simulink model "gsm_ddc_model"  (R2025a)
settings: Solver=VariableStepAuto  StartTime=0.0  StopTime=3  FixedStep=0.00005  RelTol=1e-3
undefined symbols (not defined in the file): designMultirateFIR, dspblkCoreblockFVToolHelper, gcbh
libraries: dspmlti4 x10, dspsigops x8, dspsrcs4 x8
settings Model: Creator=User  LastModifiedBy=User
settings OptimizationCC: DefaultParameterBehavior=Inlined  EnhancedBackFolding=on  PassReuseOutputArgsAs=Individual arguments  ZeroExternalMemoryAtStartup=off  ZeroInternalMemoryAtStartup=off  OptimizeBlockOrder=speed  DifferentSizesBufferReuse=on  OptimizationCustomize=off  EfficientTunableParamExpr=on
settings DebuggingCC: ParameterTunabilityLossMsg=error
settings HardwareCC: TargetBitPerPointer=64.0  TargetBitPerSizeT=64.0  TargetBitPerPtrDiffT=64.0  TargetLongLongMode=on  TargetIntDivRoundTo=Zero  TargetEndianess=LittleEndian  TargetWordSize=64.0  TargetHWDeviceType=MATLAB Host  ProdEqTarget=off
settings SFSimCC: MATLABDynamicMemAlloc=off
settings RTWCC: SystemTargetFile=ert.tlc  GenCodeOnly=on  TemplateMakefile=ert_default_tmf  Toolchain=MinGW64 | CMake/gmake (64-bit Windows)  BuildConfiguration=RelWithDebInfo  DataTypeReplacement=CDataTypesFixedWidth  TargetLang=C++  Description=Embedded Coder
settings CodeAppCC: ForceParamTrailComments=on  IgnoreCustomStorageClasses=off  OperatorAnnotations=on  SimulinkDataObjDesc=on  SFDataObjDesc=on  InsertBlockDesc=on
settings ERTTargetCC: ExtModeTransport=0.0  ExtModeStaticAlloc=off  ExtModeMexFile=ext_comm  ExtModeIntrfLevel=Level1  RootIOFormat=Structure reference  ERTCustomFileTemplate=example_file_process.tlc  MaxIdInt64=INT64_MAX  MinIdInt64=INT64_MIN  MaxIdUint64=UINT64_MAX  MaxIdInt32=INT32_MAX  MinIdInt32=INT32_MIN  MaxIdUint32=UINT32_MAX  MaxIdInt16=INT16_MAX  MinIdInt16=INT16_MIN  MaxIdUint16=UINT16_MAX  MaxIdInt8=INT8_MAX  MinIdInt8=INT8_MIN  MaxIdUint8=UINT8_MAX  TargetLangStandard=C++17 (ISO)  GenerateSampleERTMain=on  SuppressErrorStatus=on  PreserveMATLABNamespacesInGeneratedCode=off

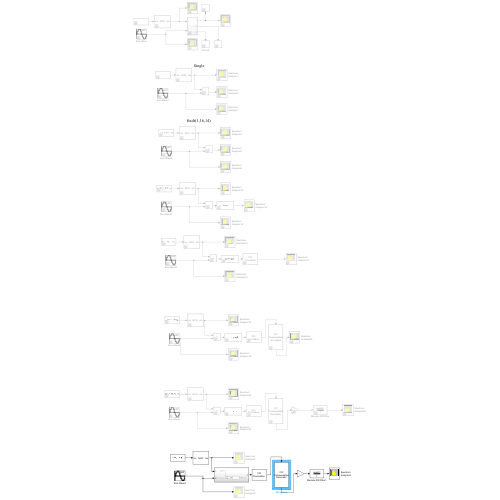
[thumbnail: Simulink's stored preview of the top-level diagram]
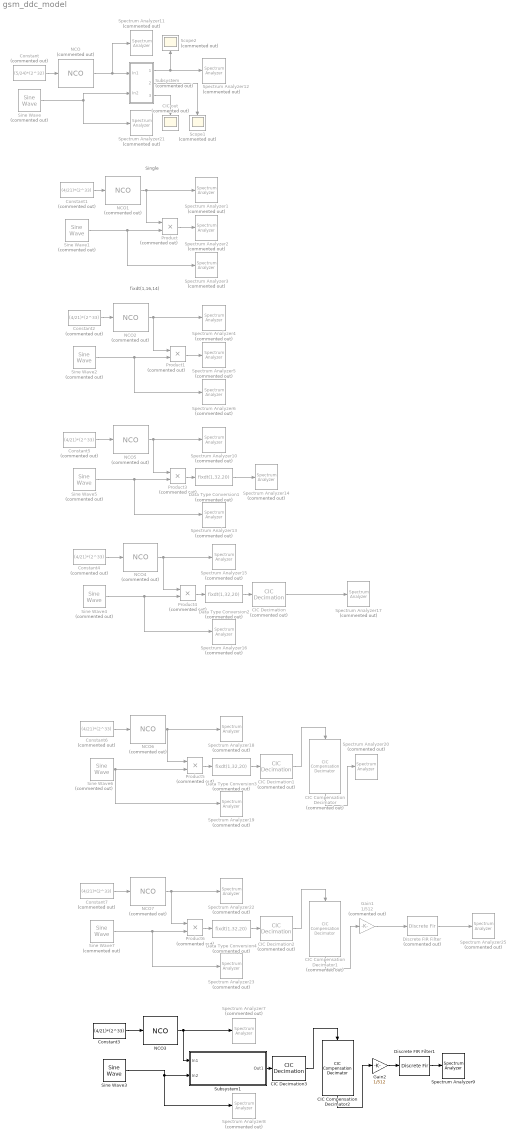
== system gsm_ddc_model ==
  note: Single
  note: fixdt(1,16,14)
  CIC Decimation : dspmlti4/CIC Decimation  Commented=on  filtFrom=Dialog parameters  filtobj=CICDECIM  ftype=Decimator  R=64  M=1  N=6  filterInternals=Minimum section word lengths  BPS=[16 16 16 16]  FLPS=0  outputWordLength=40  outputFracLength=0  launchFVT=off  framing=Maintain input frame rate  RateOptions=Allow multirate processing
  CIC Decimation1 : dspmlti4/CIC Decimation  Commented=on  filtFrom=Dialog parameters  filtobj=CICDECIM  ftype=Decimator  R=64  M=1  N=6  filterInternals=Minimum section word lengths  BPS=[16 16 16 16]  FLPS=0  outputWordLength=40  outputFracLength=0  launchFVT=off  framing=Maintain input frame rate  RateOptions=Allow multirate processing
  CIC Decimation2 : dspmlti4/CIC Decimation  Commented=on  filtFrom=Dialog parameters  filtobj=CICDECIM  ftype=Decimator  R=64  M=1  N=6  filterInternals=Minimum section word lengths  BPS=[16 16 16 16]  FLPS=0  outputWordLength=40  outputFracLength=0  launchFVT=off  framing=Maintain input frame rate  RateOptions=Allow multirate processing
  CIC Decimation3 : dspmlti4/CIC Decimation  filtFrom=Dialog parameters  filtobj=CICDECIM  ftype=Decimator  R=64  M=1  N=6  filterInternals=Minimum section word lengths  BPS=[16 16 16 16]  FLPS=0  outputWordLength=40  outputFracLength=0  launchFVT=off  framing=Maintain input frame rate  RateOptions=Allow multirate processing
  CIC Compensation Decimator : dspmlti4/CIC Compensation Decimator  Commented=on  CICRateChangeFactor=64  CICNumSections=6  CICDifferentialDelay=1  DecimationFactor=1  DesignForMinimumOrder=on  FilterOrder=12  PassbandFrequency=500000  StopbandFrequency=700000  PassbandRipple=0.1  StopbandAttenuation=60  SampleRateMode=Specify on dialog  SampleRate=122.88e6/64  AllowArbitraryInputLength=off  SimulateUsing=Code generation  roundingMode=Floor  coeffsDataTypeStr=fixdt(1,32,20)
  CIC Compensation Decimator1 : dspmlti4/CIC Compensation Decimator  Commented=on  CICRateChangeFactor=64  CICNumSections=6  CICDifferentialDelay=1  DecimationFactor=1  DesignForMinimumOrder=on  FilterOrder=12  PassbandFrequency=500000  StopbandFrequency=700000  PassbandRipple=0.1  StopbandAttenuation=60  SampleRateMode=Specify on dialog  SampleRate=122.88e6/64  AllowArbitraryInputLength=off  SimulateUsing=Code generation  roundingMode=Floor  coeffsDataTypeStr=fixdt(1,32,20)
  CIC Compensation Decimator2 : dspmlti4/CIC Compensation Decimator  CICRateChangeFactor=64  CICNumSections=6  CICDifferentialDelay=1  DecimationFactor=1  DesignForMinimumOrder=on  FilterOrder=12  PassbandFrequency=500000  StopbandFrequency=700000  PassbandRipple=0.1  StopbandAttenuation=60  SampleRateMode=Specify on dialog  SampleRate=122.88e6/64  AllowArbitraryInputLength=off  SimulateUsing=Code generation  roundingMode=Floor  coeffsDataTypeStr=fixdt(1,32,20)
  CIC out : Scope  Commented=on
  Constant : Constant  Commented=on  Value=(5/24)*(2^32)
  Constant{1,4..7} (5 alike) : Constant  Commented=on  Value=(4/21)*(2^33)  OutDataTypeStr=int64  LockScale=on
  Constant2 : Constant  Commented=on  Value=(4/21)*(2^33)  OutDataTypeStr=fixdt(0,33,0)  LockScale=on
  Constant3 : Constant  Value=(4/21)*(2^33)  OutDataTypeStr=int64  LockScale=on
  Data Type Conversion{1..4} (4 alike) : DataTypeConversion  Commented=on  OutMin=[-2]  OutMax=[2]  OutDataTypeStr=fixdt(1,32,20)  RndMeth=Nearest  SaturateOnIntegerOverflow=off  LockScale=on
  Discrete FIR Filter : DiscreteFir  Commented=on  LoadFcn=dspblkCoreblockFVToolHelper(gcbh,'load');  Coefficients="[-0.004427145357565 -0.000457730949878 0.008757022384944\t-0.006553011374012 -0.010338662303882 0.022622726639153 -0.000995294543376 -0.039144766526059 0.039316007159450 0.036601620368522 -0.118731802111263 0.050898933665675 0.522230710949693 0.522230710949693 0.050898933665675 -0.118731802111263 0.036601620368522 0.039316007159450 -0.039144766526059 -0.000995294543376 0.022622726639153 -0.010338662303882 -0.006553011374012 0.008757022384944 -0.000457730949878 -0.004427145357565]"  CoefDataTypeStr=fixdt(1,32,20)  ProductDataTypeStr=fixdt(1,32,20)  AccumDataTypeStr=fixdt(1,40,28)  OutDataTypeStr=fixdt(1,16,14)  SaturateOnIntegerOverflow=on
      settings: CopyFcn=dspblkCoreblockFVToolHelper(gcbh,'copy');  DeleteFcn=dspblkCoreblockFVToolHelper(gcbh,'close');  ModelCloseFcn=dspblkCoreblockFVToolHelper(gcbh,'close');  PreSaveFcn=dspblkCoreblockFVToolHelper(gcbh,'presave');  PostSaveFcn=dspblkCoreblockFVToolHelper(gcbh,'postsave');  CloseFcn=dspblkCoreblockFVToolHelper(gcbh,'close');
  Discrete FIR Filter1 : DiscreteFir  LoadFcn=dspblkCoreblockFVToolHelper(gcbh,'load');  Coefficients="[-0.004427145357565 -0.000457730949878 0.008757022384944\t-0.006553011374012 -0.010338662303882 0.022622726639153 -0.000995294543376 -0.039144766526059 0.039316007159450 0.036601620368522 -0.118731802111263 0.050898933665675 0.522230710949693 0.522230710949693 0.050898933665675 -0.118731802111263 0.036601620368522 0.039316007159450 -0.039144766526059 -0.000995294543376 0.022622726639153 -0.010338662303882 -0.006553011374012 0.008757022384944 -0.000457730949878 -0.004427145357565]"  CoefDataTypeStr=fixdt(1,32,20)  ProductDataTypeStr=fixdt(1,32,20)  AccumDataTypeStr=fixdt(1,40,28)  OutDataTypeStr=fixdt(1,16,14)  SaturateOnIntegerOverflow=on
      settings: CopyFcn=dspblkCoreblockFVToolHelper(gcbh,'copy');  DeleteFcn=dspblkCoreblockFVToolHelper(gcbh,'close');  ModelCloseFcn=dspblkCoreblockFVToolHelper(gcbh,'close');  PreSaveFcn=dspblkCoreblockFVToolHelper(gcbh,'presave');  PostSaveFcn=dspblkCoreblockFVToolHelper(gcbh,'postsave');  CloseFcn=dspblkCoreblockFVToolHelper(gcbh,'close');
  Gain1 : Gain  Commented=on  Gain=1/512  RndMeth=Nearest  LockScale=on
  Gain2 : Gain  Gain=1/512  RndMeth=Nearest  LockScale=on
  NCO : dspsigops/NCO  Commented=on  AccIncSrc=Input port  AccInc=100  PhaseOffsetSrc=Specify via dialog  PhaseOffset=0  AccumWL=32  HasDither=on  DitherWL=16  PNgeneratorLength=19  HasPhaseQuantizer=on  TableDepth=18  HasOutputPhaseError=off  Formula=Sine  DataType=Binary point scaling  OutputWL=16  OutputFL=14  CompMethod=Table lookup (no interpolation)  SampleTime=1  SamplesPerFrame=256  OutputFrames=off
  NCO1 : dspsigops/NCO  Commented=on  AccIncSrc=Input port  AccInc=100  PhaseOffsetSrc=Specify via dialog  PhaseOffset=0  AccumWL=33  HasDither=off  DitherWL=16  PNgeneratorLength=19  HasPhaseQuantizer=on  TableDepth=24  HasOutputPhaseError=off  Formula=Sine  DataType=single  OutputWL=16  OutputFL=14  CompMethod=Table lookup (no interpolation)  SampleTime=1  SamplesPerFrame=64  OutputFrames=off
  NCO2 : dspsigops/NCO  Commented=on  AccIncSrc=Input port  AccInc=100  PhaseOffsetSrc=Specify via dialog  PhaseOffset=0  AccumWL=33  HasDither=off  DitherWL=20  PNgeneratorLength=19  HasPhaseQuantizer=on  TableDepth=18  HasOutputPhaseError=off  Formula=Sine  DataType=Binary point scaling  OutputWL=16  OutputFL=14  CompMethod=Table lookup (no interpolation)  SampleTime=1  SamplesPerFrame=64  OutputFrames=off
  NCO3 : dspsigops/NCO  AccIncSrc=Input port  AccInc=100  PhaseOffsetSrc=Specify via dialog  PhaseOffset=0  AccumWL=33  HasDither=on  DitherWL=14  PNgeneratorLength=19  HasPhaseQuantizer=on  TableDepth=24  HasOutputPhaseError=off  Formula=Sine  DataType=single  OutputWL=16  OutputFL=14  CompMethod=Table lookup (no interpolation)  SampleTime=1  SamplesPerFrame=64  OutputFrames=off
  NCO{4..7} (4 alike) : dspsigops/NCO  Commented=on  AccIncSrc=Input port  AccInc=100  PhaseOffsetSrc=Specify via dialog  PhaseOffset=0  AccumWL=33  HasDither=on  DitherWL=14  PNgeneratorLength=19  HasPhaseQuantizer=on  TableDepth=24  HasOutputPhaseError=off  Formula=Sine  DataType=single  OutputWL=16  OutputFL=14  CompMethod=Table lookup (no interpolation)  SampleTime=1  SamplesPerFrame=64  OutputFrames=off
  Product{,3..6} (5 alike) : Product  Commented=on  InputSameDT=on  OutDataTypeStr=single  RndMeth=Nearest  SaturateOnIntegerOverflow=on
  Product1 : Product  Commented=on  InputSameDT=on  OutMin=[-2]  OutMax=[4]  OutDataTypeStr=fixdt(1,40,36)  RndMeth=Nearest  SaturateOnIntegerOverflow=on
  Scope1 : Scope  Commented=on
  Scope2 : Scope  Commented=on
      settings: DataLoggingVariableName=ScopeData2
  Sine Wave : dspsrcs4/Sine Wave  Commented=on  Amplitude=1  Frequency=100  Phase=0  SampleMode=Discrete  OutComplex=Real  CompMethod=Trigonometric fcn  TableSize=Speed  SampleTime=1/1000  SamplesPerFrame=1  ResetState=Restart at time zero  OutputFrames=off  dataType=double  wordLen=16  udDataType=sfix(16)  fracBitsMode=Best precision  numFracBits=15  OutDataTypeStr=double  LastOutDataTypeStr=double
  Sine Wave{1,4..7} (5 alike) : dspsrcs4/Sine Wave  Commented=on  Amplitude=1  Frequency=122.88e6*(4/21)  Phase=0  SampleMode=Discrete  OutComplex=Real  CompMethod=Trigonometric fcn  TableSize=Speed  SampleTime=1/122.88e6  SamplesPerFrame=64  ResetState=Restart at time zero  OutputFrames=off  dataType=single  wordLen=16  udDataType=sfix(16)  fracBitsMode=Best precision  numFracBits=15  OutDataTypeStr=single  LastOutDataTypeStr=single
  Sine Wave2 : dspsrcs4/Sine Wave  Commented=on  Amplitude=1  Frequency=1/(5/122.88e6)  Phase=0  SampleMode=Discrete  OutComplex=Real  CompMethod=Table lookup  TableSize=Speed  SampleTime=1/122.88e6  SamplesPerFrame=64  ResetState=Restart at time zero  OutputFrames=off  dataType=Fixed-point  wordLen=16  udDataType=sfix(16)  fracBitsMode=User-defined  numFracBits=14  OutDataTypeStr=fixdt(1,16,14)  LastOutDataTypeStr=fixdt(1,16,14)
  Sine Wave3 : dspsrcs4/Sine Wave  Amplitude=1  Frequency=122.88e6*(4/21)  Phase=0  SampleMode=Discrete  OutComplex=Real  CompMethod=Trigonometric fcn  TableSize=Speed  SampleTime=1/122.88e6  SamplesPerFrame=64  ResetState=Restart at time zero  OutputFrames=off  dataType=single  wordLen=16  udDataType=sfix(16)  fracBitsMode=Best precision  numFracBits=15  OutDataTypeStr=single  LastOutDataTypeStr=single
  Spectrum Analyzer1 : SpectrumAnalyzer  Commented=on  WindowPosition=[1.000000,41.000000,1536.000000,801.000000,]  ScopeFrameLocation=window  SampleRate=44.1e3  WindowInvariantSamplesPerUpdate=on  FilterSharpness=0.5  StartFrequency=20  StopFrequency=20e3  ReferenceLoad=50  YLimits=[-220.3667 32.2515]  SelectedToolstripTab=spectrumAnalyzerToolstrip.measurementsTab
  Spectrum Analyzer{7,10,15,18,22} (5 alike) : SpectrumAnalyzer  Commented=on  WindowPosition=[0.000000,32.000000,1536.000000,801.000000,]  ScopeFrameLocation=window  SampleRate=44.1e3  WindowInvariantSamplesPerUpdate=on  FilterSharpness=0.5  StartFrequency=20  StopFrequency=20e3  ReferenceLoad=50  YLimits=[-150.8801 24.5308]  SelectedToolstripTab=spectrumAnalyzerToolstrip.measurementsTab
  Spectrum Analyzer11 : SpectrumAnalyzer  Commented=on  WindowPosition=[368.000000,182.000000,800.000000,500.000000,]  ScopeFrameLocation=window  SampleRate=44.1e3  PlotAsTwoSidedSpectrum=off  FrequencyScale=Log  WindowInvariantSamplesPerUpdate=on  FrequencySpan=Start and stop frequencies  StartFrequency=20  StopFrequency=20e3
  Spectrum Analyzer12 : SpectrumAnalyzer  Commented=on  WindowPosition=[368.000000,182.000000,800.000000,500.000000,]  ScopeFrameLocation=window  SampleRate=44.1e3  PlotAsTwoSidedSpectrum=off  FrequencyScale=Log  WindowInvariantSamplesPerUpdate=on  FrequencySpan=Start and stop frequencies  StartFrequency=20  StopFrequency=20e3
  Spectrum Analyzer{8,13,16,19,23} (5 alike) : SpectrumAnalyzer  Commented=on  WindowPosition=[0.000000,32.000000,1536.000000,801.000000,]  ScopeFrameLocation=window  SampleRate=44.1e3  WindowInvariantSamplesPerUpdate=on  StartFrequency=20  StopFrequency=200000  ReferenceLoad=50  MaximizeAxes=Off  YLimits=[-205.4426 30.5933]  SelectedToolstripTab=spectrumAnalyzerToolstrip.measurementsTab
  Spectrum Analyzer14 : SpectrumAnalyzer  Commented=on  WindowPosition=[1.000000,41.000000,1536.000000,801.000000,]  ScopeFrameLocation=window  SampleRate=44.1e3  WindowInvariantSamplesPerUpdate=on  FilterSharpness=0.5  StartFrequency=20  StopFrequency=20e3  ReferenceLoad=50  YLimits=[-154.9421 23.2522]  SelectedToolstripTab=spectrumAnalyzerToolstrip.measurementsTab
  Spectrum Analyzer17 : SpectrumAnalyzer  Commented=on  WindowPosition=[1.000000,41.000000,1536.000000,801.000000,]  ScopeFrameLocation=window  SampleRate=44.1e3  WindowInvariantSamplesPerUpdate=on  FilterSharpness=0.5  StartFrequency=20  StopFrequency=20e3  ReferenceLoad=50  YLimits=[17.5809 243.7732]  SelectedToolstripTab=spectrumAnalyzerToolstrip.measurementsTab
  Spectrum Analyzer2 : SpectrumAnalyzer  Commented=on  WindowPosition=[1.000000,41.000000,1536.000000,801.000000,]  ScopeFrameLocation=window  SampleRate=44.1e3  WindowInvariantSamplesPerUpdate=on  FilterSharpness=0.5  StartFrequency=20  StopFrequency=20e3  ReferenceLoad=50  MaximizeAxes=Off  YLimits=[-203.0353 23.6363]  SelectedToolstripTab=spectrumAnalyzerToolstrip.estimationTab
  Spectrum Analyzer20 : SpectrumAnalyzer  Commented=on  WindowPosition=[1.000000,41.000000,1536.000000,801.000000,]  ScopeFrameLocation=window  SampleRate=44.1e3  WindowInvariantSamplesPerUpdate=on  FilterSharpness=0.5  StartFrequency=20  StopFrequency=20e3  ReferenceLoad=50  YLimits=[4.3785 247.9779]  SelectedToolstripTab=spectrumAnalyzerToolstrip.measurementsTab
  Spectrum Analyzer21 : SpectrumAnalyzer  Commented=on  WindowPosition=[560.000000,350.000000,800.000000,500.000000,]  ScopeFrameLocation=window  SampleRate=44.1e3  PlotAsTwoSidedSpectrum=off  FrequencyScale=Log  WindowInvariantSamplesPerUpdate=on  FrequencySpan=Start and stop frequencies  StartFrequency=20  StopFrequency=20e3
  Spectrum Analyzer25 : SpectrumAnalyzer  Commented=on  WindowPosition=[1.000000,41.000000,1536.000000,801.000000,]  ScopeFrameLocation=window  SampleRate=44.1e3  WindowInvariantSamplesPerUpdate=on  FilterSharpness=0.5  StartFrequency=20  StopFrequency=20e3  ReferenceLoad=50  YLimits=[-204.1761 43.8317]  SelectedToolstripTab=spectrumAnalyzerToolstrip.channelMeasurementsTab
  Spectrum Analyzer3 : SpectrumAnalyzer  Commented=on  WindowPosition=[1.000000,41.000000,1536.000000,801.000000,]  ScopeFrameLocation=window  SampleRate=44.1e3  WindowInvariantSamplesPerUpdate=on  StartFrequency=20  StopFrequency=200000  ReferenceLoad=50  MaximizeAxes=Off  YLimits=[-204.6783 30.5084]  SelectedToolstripTab=spectrumAnalyzerToolstrip.measurementsTab
  Spectrum Analyzer4 : SpectrumAnalyzer  Commented=on  WindowPosition=[1.000000,41.000000,1536.000000,801.000000,]  ScopeFrameLocation=window  SampleRate=44.1e3  WindowInvariantSamplesPerUpdate=on  FilterSharpness=0.5  StartFrequency=20  StopFrequency=20e3  ReferenceLoad=50  YLimits=[-166.5076 26.2672]  SelectedToolstripTab=spectrumAnalyzerToolstrip.measurementsTab
  Spectrum Analyzer5 : SpectrumAnalyzer  Commented=on  WindowPosition=[1.000000,41.000000,1536.000000,801.000000,]  ScopeFrameLocation=window  SampleRate=44.1e3  WindowInvariantSamplesPerUpdate=on  FilterSharpness=0.5  StartFrequency=20  StopFrequency=20e3  ReferenceLoad=50  MaximizeAxes=Off  YLimits=[-165.2004 19.4324]  SelectedToolstripTab=spectrumAnalyzerToolstrip.measurementsTab
  Spectrum Analyzer6 : SpectrumAnalyzer  Commented=on  WindowPosition=[0.000000,42.000000,1536.000000,793.000000,]  ScopeFrameLocation=window  SampleRate=44.1e3  WindowInvariantSamplesPerUpdate=on  StartFrequency=20  StopFrequency=200000  ReferenceLoad=50  MaximizeAxes=Off  YLimits=[-281.436 39.0316]  SelectedToolstripTab=spectrumAnalyzerToolstrip.measurementsTab
  Spectrum Analyzer9 : SpectrumAnalyzer  WindowPosition=[1.000000,41.000000,1536.000000,801.000000,]  ScopeFrameLocation=window  SampleRate=44.1e3  WindowInvariantSamplesPerUpdate=on  FilterSharpness=0.5  StartFrequency=20  StopFrequency=20e3  ReferenceLoad=50  YLimits=[-204.1761 43.8317]  SelectedToolstripTab=spectrumAnalyzerToolstrip.channelMeasurementsTab
  Subsystem : Subsystem  Commented=on
  Subsystem1 : Subsystem
  wires:
  NCO/1 -> Subsystem/1(In1), Spectrum Analyzer11/1
  Constant/1 -> NCO/1
  Sine Wave/1 -> Spectrum Analyzer21/1, Subsystem/2(In2)
  Subsystem/2(Out2) -> Scope1/1
  Subsystem/3(Out3) -> CIC out/1
  Subsystem/1(Out1) -> Spectrum Analyzer12/1, Scope2/1
  Constant1/1 -> NCO1/1
  NCO1/1 -> Spectrum Analyzer1/1, Product/1
  Sine Wave1/1 -> Spectrum Analyzer3/1, Product/2
  Product/1 -> Spectrum Analyzer2/1
  NCO2/1 -> Spectrum Analyzer4/1, Product1/1
  Sine Wave2/1 -> Spectrum Analyzer6/1, Product1/2
  Constant2/1 -> NCO2/1
  Product1/1 -> Spectrum Analyzer5/1
  Product3/1 -> Data Type Conversion1/1
  NCO5/1 -> Product3/1, Spectrum Analyzer10/1
  Sine Wave5/1 -> Product3/2, Spectrum Analyzer13/1
  Constant5/1 -> NCO5/1
  Data Type Conversion1/1 -> Spectrum Analyzer14/1
  NCO4/1 -> Product4/1, Spectrum Analyzer15/1
  Constant4/1 -> NCO4/1
  Sine Wave4/1 -> Product4/2, Spectrum Analyzer16/1
  Product4/1 -> Data Type Conversion2/1
  Data Type Conversion2/1 -> CIC Decimation/1
  CIC Decimation/1 -> Spectrum Analyzer17/1
  Data Type Conversion3/1 -> CIC Decimation1/1
  Sine Wave6/1 -> Product5/2, Spectrum Analyzer19/1
  Product5/1 -> Data Type Conversion3/1
  Constant6/1 -> NCO6/1
  NCO6/1 -> Product5/1, Spectrum Analyzer18/1
  CIC Decimation1/1 -> CIC Compensation Decimator/1
  CIC Compensation Decimator/1 -> Spectrum Analyzer20/1
  Constant7/1 -> NCO7/1
  CIC Decimation2/1 -> CIC Compensation Decimator1/1
  CIC Compensation Decimator1/1 -> Gain1/1
  NCO7/1 -> Product6/1, Spectrum Analyzer22/1
  Sine Wave7/1 -> Product6/2, Spectrum Analyzer23/1
  Data Type Conversion4/1 -> CIC Decimation2/1
  Product6/1 -> Data Type Conversion4/1
  Gain1/1 -> Discrete FIR Filter/1
  Discrete FIR Filter/1 -> Spectrum Analyzer25/1
  Gain2/1 -> Discrete FIR Filter1/1
  Sine Wave3/1 -> Subsystem1/2(In2), Spectrum Analyzer8/1
  CIC Compensation Decimator2/1 -> Gain2/1
  Constant3/1 -> NCO3/1
  CIC Decimation3/1 -> CIC Compensation Decimator2/1
  Discrete FIR Filter1/1 -> Spectrum Analyzer9/1
  NCO3/1 -> Subsystem1/1(In1), Spectrum Analyzer7/1
  Subsystem1/1(Out1) -> CIC Decimation3/1

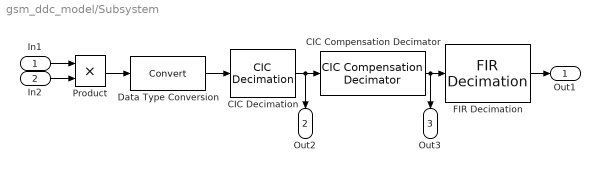
== system gsm_ddc_model/Subsystem ==
  In1 : Inport
  In2 : Inport  Port=2
  CIC Decimation : dspmlti4/CIC Decimation  filtFrom=Dialog parameters  filtobj=CICDECIM  ftype=Decimator  R=2  M=1  N=2  filterInternals=Full precision  BPS=[16 16 16 16]  FLPS=0  outputWordLength=32  outputFracLength=0  launchFVT=off  framing=Maintain input frame rate  RateOptions=Enforce single-rate processing
  CIC Compensation Decimator : dspmlti4/CIC Compensation Decimator  CICRateChangeFactor=2  CICNumSections=2  CICDifferentialDelay=1  DecimationFactor=2  DesignForMinimumOrder=on  FilterOrder=12  PassbandFrequency=0.16667  StopbandFrequency=0.66667  PassbandRipple=0.1  StopbandAttenuation=60  SampleRateMode=Use normalized frequency (0 to 1)  SampleRate=1200000  AllowArbitraryInputLength=off  SimulateUsing=Interpreted execution  roundingMode=Floor  coeffsDataTypeStr=fixdt(1,16)
  Data Type Conversion : DataTypeConversion  SaturateOnIntegerOverflow=off  RndMeth=Floor
  FIR Decimation : dspmlti4/FIR Decimation  FilterSource=Auto  h=designMultirateFIR(1,2)  D=2  filtStruct=Direct form  FilterObject=FDECIM  InputProcessing=Columns as channels (frame based)  framing=Enforce single-rate processing  AllowArbitraryInputLength=off  inputOffset=0  outputBufInitCond=0  roundingMode=Floor  overflowMode=off  firstCoeffDataTypeStr=Inherit: Same word length as input  firstCoeffMin=[]  firstCoeffMax=[]  firstCoeffLastDataTypeStr=Inherit: Same word length as input  outputDataTypeStr=Inherit: Same as accumulator  outputMin=[]  outputMax=[]  outputLastDataTypeStr=Inherit: Same as accumulator
  Product : Product
  Out1 : Outport
  Out2 : Outport  Port=2
  Out3 : Outport  Port=3
  wires:
  Data Type Conversion/1 -> CIC Decimation/1
  CIC Decimation/1 -> Out2/1, CIC Compensation Decimator/1
  Product/1 -> Data Type Conversion/1
  In2/1 -> Product/2
  CIC Compensation Decimator/1 -> Out3/1, FIR Decimation/1
  In1/1 -> Product/1
  FIR Decimation/1 -> Out1/1

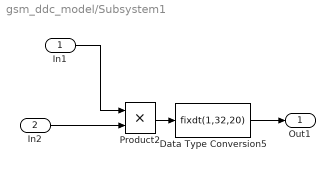
== system gsm_ddc_model/Subsystem1 ==
  In1 : Inport
  In2 : Inport  Port=2
  Data Type Conversion5 : DataTypeConversion  OutMin=[-2]  OutMax=[2]  OutDataTypeStr=fixdt(1,32,20)  RndMeth=Nearest  SaturateOnIntegerOverflow=off  LockScale=on
  Product2 : Product  InputSameDT=on  OutDataTypeStr=single  RndMeth=Nearest  SaturateOnIntegerOverflow=on
  Out1 : Outport
  wires:
  Product2/1 -> Data Type Conversion5/1
  Data Type Conversion5/1 -> Out1/1
  In1/1 -> Product2/1
  In2/1 -> Product2/2
